simulink model "quadrotor_controller"  (Simulink 7.6)
settings: Solver=FixedStepDiscrete  StartTime=0.0  StopTime=inf  FixedStep=1/100  RelTol=1e-3
InitFcn:
  | N_to_Npercent = 1/8;
  | L=0.20;
  | Ts=0.01;
settings Model: Creator=jonathan  LastModifiedBy=jonathan  SimulationMode=external
settings DataIOCC: LimitDataPoints=off
settings OptimizationCC: OptimizeModelRefInitCode=on  LifeSpan=1
settings HardwareCC: ProdBitPerLong=64  ProdLargestAtomicInteger=Long  ProdLargestAtomicFloat=Double  ProdHWDeviceType=Generic->Custom  TargetLargestAtomicInteger=Long  TargetLargestAtomicFloat=Double  TargetIntDivRoundTo=Zero  TargetEndianess=LittleEndian  TargetHWDeviceType=Generic->32-bit x86 compatible
settings RTWCC: SystemTargetFile=ert.tlc  GenCodeOnly=on  TemplateMakefile=ert_default_tmf  PostCodeGenCommand=packNGo (buildInfo);  Description=Real-Time Workshop Embedded Coder  ProcessScript=ert_make_rtw_hook  TargetLang=C++  RTWCompilerOptimization=On
settings CodeAppCC: IgnoreCustomStorageClasses=off
settings ERTTargetCC: MultiwordLength=2048  GeneratePreprocessorConditionals=Enable all  ExtMode=on  ExtModeMexArgs='127.0.0.1'  ERTCustomFileTemplate=example_file_process.tlc  ConvertIfToSwitch=off

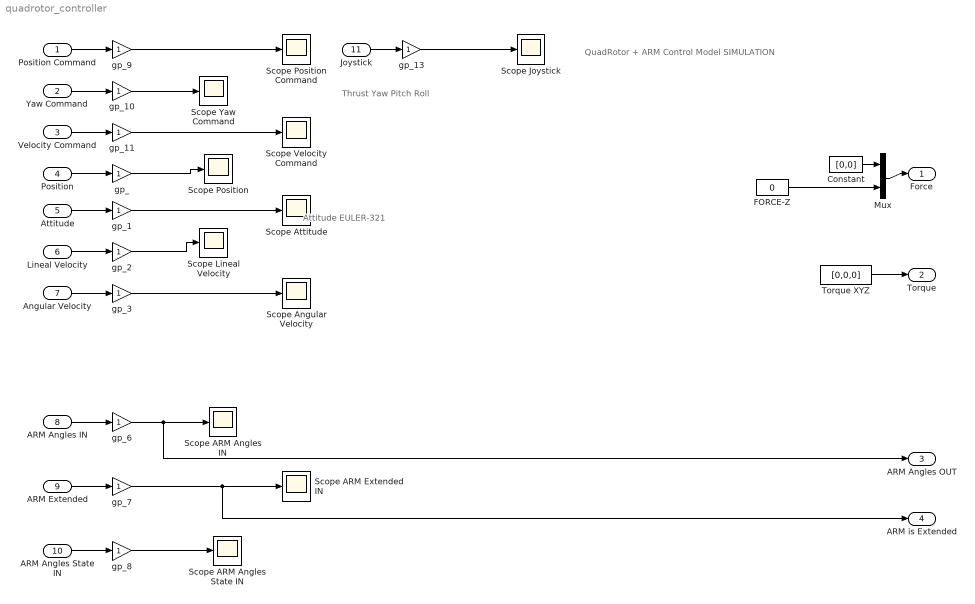
== system quadrotor_controller ==
  note: QuadRotor + ARM
      | Control Model
      | SIMULATION
  note: Thrust
      | Yaw
      | Pitch
      | Roll
  note: Attitude
      | EULER-321
  Position Command : Inport  OutDataTypeStr=double  PortDimensions=3
  Yaw Command : Inport  Port=2  OutDataTypeStr=double  PortDimensions=1
  Velocity Command : Inport  Port=3  OutDataTypeStr=double  PortDimensions=1
  Position : Inport  Port=4  OutDataTypeStr=double  PortDimensions=3
  Attitude : Inport  Port=5  OutDataTypeStr=double  PortDimensions=3
  Lineal Velocity : Inport  Port=6  OutDataTypeStr=double  PortDimensions=3
  Angular Velocity : Inport  Port=7  OutDataTypeStr=double  PortDimensions=3
  ARM Angles IN : Inport  Port=8  OutDataTypeStr=double  PortDimensions=8
  ARM Extended : Inport  Port=9  OutDataTypeStr=double  PortDimensions=1
  ARM Angles State IN : Inport  Port=10  OutDataTypeStr=double  PortDimensions=8
  Joystick : Inport  Port=11  OutDataTypeStr=double  PortDimensions=4
  Constant : Constant  Value=[0,0]
  FORCE-Z : Constant  Value=0
  Mux : Mux  Inputs=2
  Scope ARM Angles State IN : Scope
      settings: SaveName=ScopeData8
  Scope ARM Angles IN : Scope
      settings: SaveName=ScopeData6
  Scope ARM Extended IN : Scope
      settings: SaveName=ScopeData7
  Scope Angular Velocity : Scope
      settings: YMin=-0.45  YMax=0.5  SaveName=ScopeData3
  Scope Attitude : Scope
      settings: YMin=-0.9  YMax=0.6
  Scope Joystick : Scope
      settings: YMin=-1  YMax=1  SaveName=ScopeData13
  Scope Lineal Velocity : Scope
      settings: YMin=-0.15  YMax=0.2  SaveName=ScopeData2
  Scope Position : Scope
      settings: YMin=-3  YMax=11
  Scope Position Command : Scope
      settings: SaveName=ScopeData9
  Scope Velocity Command : Scope
      settings: SaveName=ScopeData11
  Scope Yaw Command : Scope
      settings: SaveName=ScopeData10
  Torque XYZ : Constant  Value=[0,0,0]
  gp_{,1..3,6,8..11,13} (10 alike) : Gain
  gp_7 : Gain  OutDataTypeStr=Inherit: Same as input
  Force : Outport  OutDataTypeStr=double  PortDimensions=3
  Torque : Outport  Port=2  OutDataTypeStr=double  PortDimensions=3
  ARM Angles OUT : Outport  Port=3  OutDataTypeStr=double  PortDimensions=8
  ARM is Extended : Outport  Port=4  OutDataTypeStr=double  PortDimensions=1
  wires:
  Position/1 -> gp_/1
  Attitude/1 -> gp_1/1
  Lineal Velocity/1 -> gp_2/1
  Angular Velocity/1 -> gp_3/1
  ARM Extended/1 -> gp_7/1
  ARM Angles IN/1 -> gp_6/1
  gp_/1 -> Scope Position/1
  gp_1/1 -> Scope Attitude/1
  gp_2/1 -> Scope Lineal Velocity/1
  gp_3/1 -> Scope Angular Velocity/1
  gp_6/1 -> Scope ARM Angles IN/1, ARM Angles OUT/1
  gp_7/1 -> Scope ARM Extended IN/1, ARM is Extended/1
  ARM Angles State IN/1 -> gp_8/1
  gp_8/1 -> Scope ARM Angles State IN/1
  Constant/1 -> Mux/1
  Mux/1 -> Force/1
  Position Command/1 -> gp_9/1
  gp_9/1 -> Scope Position Command/1
  Yaw Command/1 -> gp_10/1
  gp_10/1 -> Scope Yaw Command/1
  Velocity Command/1 -> gp_11/1
  gp_11/1 -> Scope Velocity Command/1
  Joystick/1 -> gp_13/1
  gp_13/1 -> Scope Joystick/1
  Torque XYZ/1 -> Torque/1
  FORCE-Z/1 -> Mux/2
